simulink model "yanshou51"  (R2017a)
settings: Solver=VariableStepAuto  StartTime=0.0  StopTime=10.0  RelTol=1e-3
settings Model: Creator=adi  LastModifiedBy=adi

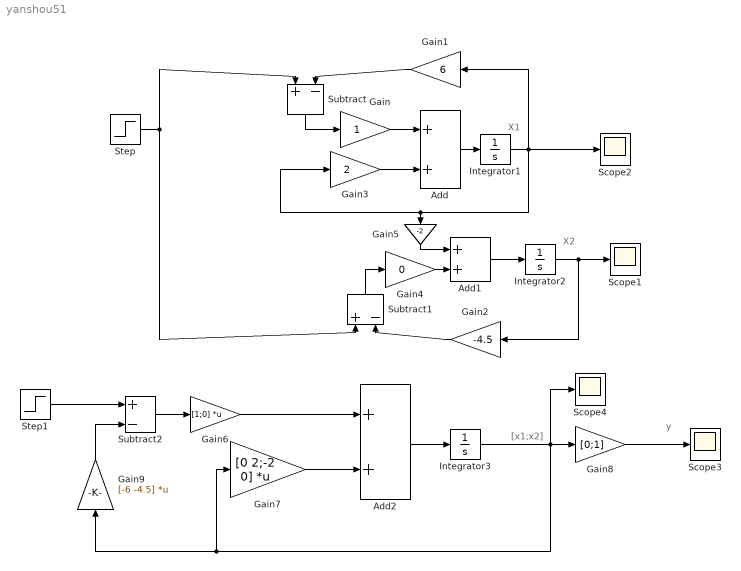
== system yanshou51 ==
  note: y
  note: [x1;x2]
  note: X2
  note: X1
  Add : Sum
  Add1 : Sum
  Add2 : Sum
  Gain : Gain
  Gain1 : Gain  Gain=6
  Gain2 : Gain  Gain=-4.5
  Gain3 : Gain  Gain=2
  Gain4 : Gain  Gain=0
  Gain5 : Gain  Gain=-2
  Gain6 : Gain  Gain=[1;0]  Multiplication=Matrix(K*u)
  Gain7 : Gain  Gain=[0 2;-2 0]  Multiplication=Matrix(K*u)
  Gain8 : Gain  Gain=[0;1]
  Gain9 : Gain  Gain=[-6 -4.5]  Multiplication=Matrix(K*u)
  Integrator1 : Integrator
  Integrator2 : Integrator
  Integrator3 : Integrator
  Scope{1..4} (4 alike) : Scope
  Step : Step  SampleTime=0
  Step1 : Step  SampleTime=0
  Subtract : Sum  Inputs=+-
  Subtract1 : Sum  Inputs=+-
  Subtract2 : Sum  Inputs=+-
  wires:
  Step/1 -> Subtract/1, Subtract1/1
  Gain3/1 -> Add/2
  Add/1 -> Integrator1/1
  Gain5/1 -> Add1/1
  Add1/1 -> Integrator2/1
  Integrator1/1 -> Scope2/1, Gain5/1, Gain3/1, Gain1/1
  Integrator2/1 -> Gain2/1, Scope1/1
  Gain2/1 -> Subtract1/2
  Gain7/1 -> Add2/2
  Add2/1 -> Integrator3/1
  Integrator3/1 -> Scope4/1, Gain9/1, Gain7/1, Gain8/1
  Gain8/1 -> Scope3/1
  Gain9/1 -> Subtract2/2
  Step1/1 -> Subtract2/1
  Subtract2/1 -> Gain6/1
  Gain6/1 -> Add2/1
  Subtract1/1 -> Gain4/1
  Gain4/1 -> Add1/2
  Gain1/1 -> Subtract/2
  Gain/1 -> Add/1
  Subtract/1 -> Gain/1
